simulink model "linearized_manifold"  (Simulink 8.3)
settings: Solver=ode3  StartTime=0.0  StopTime=10.0  RelTol=1e-3
values from neighbouring files (symbols this model uses):
  A_n = T_x^-1 * linear_manifold.a * T_x    [manifold_optimisation.m]
  B_n = T_x^-1 * linear_manifold.b * T_u    [manifold_optimisation.m]
  C_n = T_y^-1 * linear_manifold.c * T_x    [manifold_optimisation.m]
  D_n = T_y^-1 * linear_manifold.d * T_u    [manifold_optimisation.m]
  mdot_in_nominal = 0.01    [manifold_optimisation.m]
  Pe = 8.36 * 10^4    (= 83600)    [InitPar.m]
  theta_in = 295    [InitPar.m]
  x_nominal = x(end,:)    [manifold_optimisation.m]
settings Model: Creator=daniel  LastModifiedBy=daniel
settings DataIOCC: SignalLoggingSaveFormat=Dataset
settings DebuggingCC: UnderspecifiedInitializationDetection=Simplified  StateNameClashWarn=none
settings GRTTargetCC: CombineOutputUpdateFcns=on  GRTInterface=off

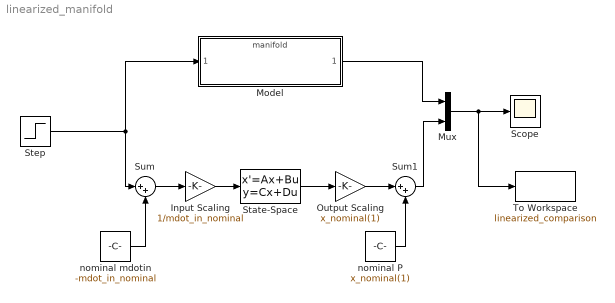
== system linearized_manifold ==
  Input Scaling : Gain  Gain=1/mdot_in_nominal
  Model : ModelReference  ModelNameDialog=manifold.mdl  SimulationMode=Normal  ModelReferenceVersion=1.22  CopyOfModelName=manifold.mdl  DefaultDataLogging=on
  Mux : Mux  Inputs=2
  "Output Scaling " : Gain  Gain=x_nominal(1)
  Scope : Scope
  State-Space : StateSpace  A=A_n  B=B_n  C=C_n  D=D_n  X0=([Pe, theta_in]-x_nominal)./x_nominal
  Step : Step  Before=0.005  After=0.015  SampleTime=0
  Sum : Sum  Inputs=|++
  Sum1 : Sum  Inputs=|++
  To Workspace : ToWorkspace  VariableName=linearized_comparison  SaveFormat=Timeseries  SampleTime=-1
  nominal P : Constant  Value=x_nominal(1)
  nominal mdotin : Constant  Value=-mdot_in_nominal
  wires:
  Step/1 -> Sum/1, Model/1
  Sum/1 -> Input Scaling/1
  nominal mdotin/1 -> Sum/2
  Model/1 -> Mux/1
  Sum1/1 -> Mux/2
  nominal P/1 -> Sum1/2
  Input Scaling/1 -> State-Space/1
  State-Space/1 -> "Output Scaling "/1
  "Output Scaling "/1 -> Sum1/1
  Mux/1 -> To Workspace/1, Scope/1
